simulink model "Control_Algo"  (R2020a)
settings: Solver=VariableStepAuto  StartTime=0.0  StopTime=10.0  RelTol=1e-3
model workspace (MAT data in the model file):
  mot.max_trq = 135
  mot.max_pwr = 38
  mot.spd = [370 739.166666667 1108.33333333 1477.5 1846.66666667 2215.83333333 2585 2954.16666667 3323.33333333 3692.5 4061.66666667 4430.83333333 4800]
  mot.trq = [135 135 135 135 135 135 130 125 120 90 80 72 65]
  mot.trq_cp = [120 112.169118269 105.297671501 99.2195136541 93.8047673037 88.9504392721 84.5738066939 80.6076640699 76.9968477689 73.6956545886 70.6658970819 90.4670202838 85.9436692696 81.8511135901 78.1306084269 74.7336254518 71.6197243914 68.7549354157]
  mot.mapL.spdindex = [100 200 300 400 500 600 700 800 900 1000 1100 1200 1300 1400 1500 1600 1700 1800 1900 2000 2100 2200 2300 2400 2500 2600 2700 2800 2900 3000 3100 3200 3300 3400 3500 3600 3700 3800 3900 4000 4100 4200 4300 4400 4500 4600 4700 4800]
  mot.mapL.trqindex = [7.5 15 22.5 30 37.5 45 52.5 60 67.5 75 82.5 90 97.5 105 112.5]
  mot.mapL.eff = [23.367031145 28.3093935 27.900833785 23.94351616 23.192960095 18.35774057 20.08454116 17.944414665 15.71176136 14.08332132 13.191387315 11.66605693 ... (720 elements, 15x48)]
  mot.mapR.spdindex = [100 200 300 400 500 600 700 800 900 1000 1100 1200 1300 1400 1500 1600 1700 1800 1900 2000 2100 2200 2300 2400 2500 2600 2700 2800 2900 3000 3100 3200 3300 3400 3500 3600 3700 3800 3900 4000 4100 4200 4300 4400 4500 4600 4700 4800]
  mot.mapR.trqindex = [7.5 15 22.5 30 37.5 45 52.5 60 67.5 75 82.5 90 97.5 105 112.5]
  mot.mapR.eff = [28.48167539 36.0807345 35.29712042 34.7163836 33.02727304 31.53442549 31.60094145 28.55014096 26.94374363 27.02005929 24.78971019 24.19758491 ... (720 elements, 15x48)]
settings Model: Creator=Administrator  LastModifiedBy=Administrator

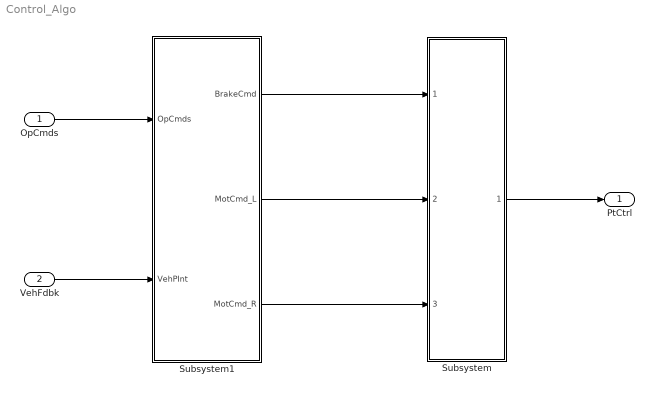
== system Control_Algo ==
  OpCmds : Inport
  VehFdbk : Inport  Port=2
  Subsystem : Subsystem
  Subsystem1 : Subsystem
  PtCtrl : Outport
  wires:
  OpCmds/1 -> Subsystem1/1(OpCmds)
  VehFdbk/1 -> Subsystem1/2(VehPInt)
  Subsystem1/1(BrakeCmd) -> Subsystem/1(BrakeCmd)
  Subsystem1/2(MotCmd_L) -> Subsystem/2(MotCmd_L)
  Subsystem1/3(MotCmd_R) -> Subsystem/3(MotCmd_R)
  Subsystem/1(OpCmd) -> PtCtrl/1

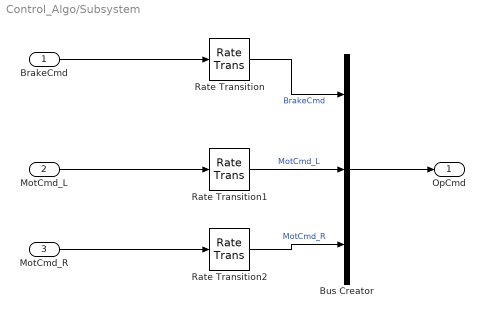
== system Control_Algo/Subsystem ==
  BrakeCmd : Inport
  MotCmd_L : Inport  Port=2
  MotCmd_R : Inport  Port=3
  Bus Creator : BusCreator  Inputs=3
  Rate Transition : RateTransition
  Rate Transition1 : RateTransition
  Rate Transition2 : RateTransition
  OpCmd : Outport
  wires:
  BrakeCmd/1 -> Rate Transition/1
  MotCmd_L/1 -> Rate Transition1/1
  MotCmd_R/1 -> Rate Transition2/1
  Rate Transition/1 -> Bus Creator/1  "BrakeCmd"
  Rate Transition1/1 -> Bus Creator/2  "MotCmd_L"
  Rate Transition2/1 -> Bus Creator/3  "MotCmd_R"
  Bus Creator/1 -> OpCmd/1

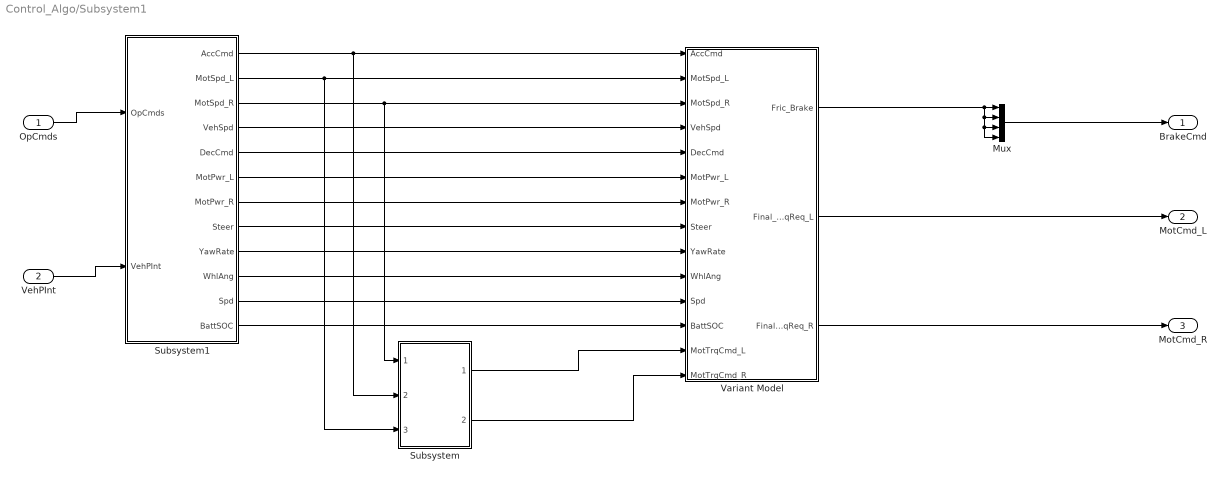
== system Control_Algo/Subsystem1 ==
  OpCmds : Inport
  VehPInt : Inport  Port=2
  Mux : Mux
  Subsystem : Subsystem
  Subsystem1 : Subsystem
  Variant Model : Subsystem  Variant=on
  BrakeCmd : Outport
  MotCmd_L : Outport  Port=2
  MotCmd_R : Outport  Port=3
  wires:
  Mux/1 -> BrakeCmd/1
  OpCmds/1 -> Subsystem1/1(OpCmds)
  VehPInt/1 -> Subsystem1/2(VehPInt)
  Subsystem1/1(AccCmd) -> Subsystem/2(AccCmd), Variant Model/1(AccCmd)
  Subsystem1/10(WhlAng) -> Variant Model/10(WhlAng)
  Subsystem1/11(Spd) -> Variant Model/11(Spd)
  Subsystem1/8(Steer) -> Variant Model/8(Steer)
  Subsystem1/9(YawRate) -> Variant Model/9(YawRate)
  Subsystem1/2(MotSpd_L) -> Subsystem/3(MotSpd_L), Variant Model/2(MotSpd_L)
  Subsystem1/3(MotSpd_R) -> Subsystem/1(MotSpd_R), Variant Model/3(MotSpd_R)
  Subsystem1/4(VehSpd) -> Variant Model/4(VehSpd)
  Subsystem1/5(DecCmd) -> Variant Model/5(DecCmd)
  Subsystem1/6(MotPwr_L) -> Variant Model/6(MotPwr_L)
  Subsystem1/7(MotPwr_R) -> Variant Model/7(MotPwr_R)
  Subsystem1/12(BattSOC) -> Variant Model/12(BattSOC)
  Subsystem/1(MotTrqCmd_L) -> Variant Model/13(MotTrqCmd_L)
  Subsystem/2(MotTrqCmd_R) -> Variant Model/14(MotTrqCmd_R)
  Variant Model/3(Final_MotTrqReq_R) -> MotCmd_R/1
  Variant Model/2(Final_MotTrqReq_L) -> MotCmd_L/1
  Variant Model/1(Fric_Brake) -> Mux/4, Mux/3, Mux/2, Mux/1

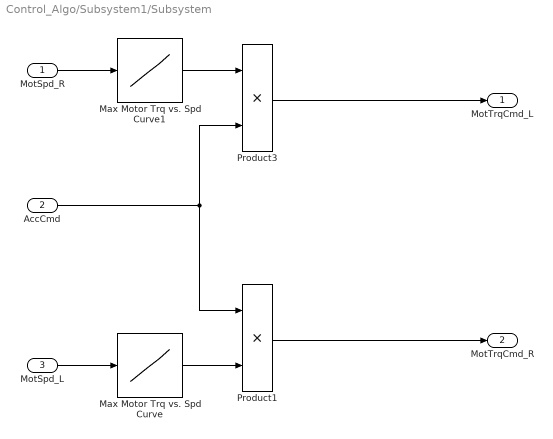
== system Control_Algo/Subsystem1/Subsystem ==
  MotSpd_R : Inport
  AccCmd : Inport  Port=2
  MotSpd_L : Inport  Port=3
  Max Motor Trq vs. Spd Curve : Lookup_n-D  NumberOfTableDimensions=1  BreakpointsForDimension1=mot.spd  Table=mot.trq  ExtrapMethod=Clip  UseLastTableValue=on  InternalRulePriority=Speed  OutDataTypeStr=Inherit: Inherit from 'Table data'  RndMeth=Simplest  InputSameDT=on
  Max Motor Trq vs. Spd Curve1 : Lookup_n-D  NumberOfTableDimensions=1  BreakpointsForDimension1=mot.spd  Table=mot.trq  ExtrapMethod=Clip  UseLastTableValue=on  InternalRulePriority=Speed  OutDataTypeStr=Inherit: Inherit from 'Table data'  RndMeth=Simplest  InputSameDT=on
  Product1 : Product
  Product3 : Product
  MotTrqCmd_L : Outport
  MotTrqCmd_R : Outport  Port=2
  wires:
  AccCmd/1 -> Product1/1, Product3/2
  Product3/1 -> MotTrqCmd_L/1
  Product1/1 -> MotTrqCmd_R/1
  Max Motor Trq vs. Spd Curve1/1 -> Product3/1
  Max Motor Trq vs. Spd Curve/1 -> Product1/2
  MotSpd_L/1 -> Max Motor Trq vs. Spd Curve/1
  MotSpd_R/1 -> Max Motor Trq vs. Spd Curve1/1

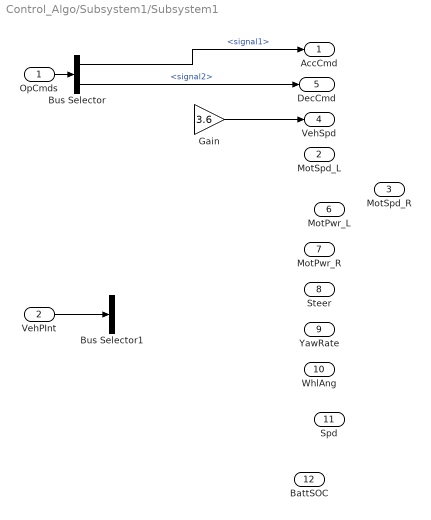
== system Control_Algo/Subsystem1/Subsystem1 ==
  OpCmds : Inport
  VehPInt : Inport  Port=2
  Bus Selector : BusSelector  OutputSignals=signal1,signal2
  Bus Selector1 : BusSelector  OutputSignals=signal1,signal2
  Gain : Gain  Gain=3.6
  AccCmd : Outport
  MotSpd_L : Outport  Port=2
  MotSpd_R : Outport  Port=3
  VehSpd : Outport  Port=4
  DecCmd : Outport  Port=5
  MotPwr_L : Outport  Port=6
  MotPwr_R : Outport  Port=7
  Steer : Outport  Port=8
  YawRate : Outport  Port=9
  WhlAng : Outport  Port=10
  Spd : Outport  Port=11
  BattSOC : Outport  Port=12
  wires:
  Bus Selector/2 -> DecCmd/1  "<signal2>"
  OpCmds/1 -> Bus Selector/1
  Bus Selector/1 -> AccCmd/1  "<signal1>"
  VehPInt/1 -> Bus Selector1/1
  Gain/1 -> VehSpd/1

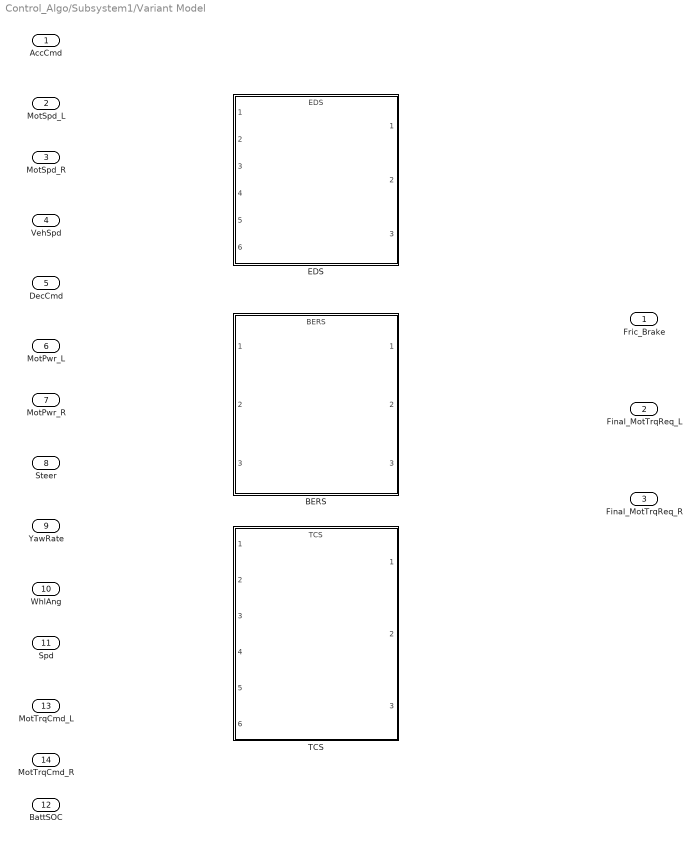
== system Control_Algo/Subsystem1/Variant Model ==
  AccCmd : Inport
  MotSpd_L : Inport  Port=2
  MotSpd_R : Inport  Port=3
  VehSpd : Inport  Port=4
  DecCmd : Inport  Port=5
  MotPwr_L : Inport  Port=6
  MotPwr_R : Inport  Port=7
  Steer : Inport  Port=8
  YawRate : Inport  Port=9
  WhlAng : Inport  Port=10
  Spd : Inport  Port=11
  BattSOC : Inport  Port=12
  MotTrqCmd_L : Inport  Port=13
  MotTrqCmd_R : Inport  Port=14
  BERS : ModelReference  ModelNameDialog=BERS.slx  VariantControl=Variant1  ModelReferenceVersion=1.2
  EDS : ModelReference  DisableCoverage=on  ModelNameDialog=EDS.slx  VariantControl=Variant  ModelReferenceVersion=1.4
  TCS : ModelReference  ModelNameDialog=TCS.slx  VariantControl=Choice  ModelReferenceVersion=1.3
  Fric_Brake : Outport
  Final_MotTrqReq_L : Outport  Port=2
  Final_MotTrqReq_R : Outport  Port=3
